simulink model "StateflowFactorial"  (R2016a)
settings: Solver=FixedStepDiscrete  StartTime=0.0  StopTime=10.0  RelTol=1e-3
settings Model: Creator=Mohamed Fawzy  LastModifiedBy=Mohamed Fawzy
settings OptimizationCC: DefaultParameterBehavior=Inlined  OptimizeModelRefInitCode=on  LifeSpan=1
settings RTWCC: SystemTargetFile=ert.tlc  GenCodeOnly=on  GenerateMakefile=off  TemplateMakefile=ert_default_tmf  GenerateReport=on  IncludeHyperlinkInReport=on  LaunchReport=on  GenerateTraceInfo=on  GenerateTraceReport=on  GenerateTraceReportSl=on  GenerateTraceReportSf=on  GenerateTraceReportEml=on
settings CodeAppCC: ForceParamTrailComments=on  IgnoreCustomStorageClasses=off  OperatorAnnotations=on  SimulinkDataObjDesc=on  SFDataObjDesc=on  MATLABFcnDesc=on  InsertBlockDesc=on  MATLABSourceComments=on
settings ERTTargetCC: GenerateSampleERTMain=on  SuppressErrorStatus=on  InlinedParameterPlacement=NonHierarchical  ERTCustomFileTemplate=example_file_process.tlc

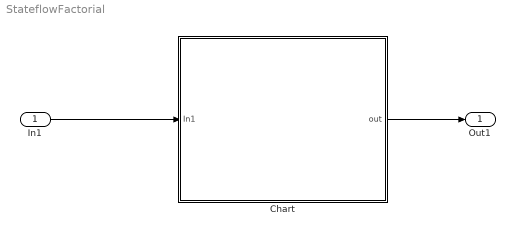
== system StateflowFactorial ==
  In1 : Inport  OutDataTypeStr=uint8
  Chart : Stateflow chart  TreatAsAtomicUnit=on
  Out1 : Outport  OutDataTypeStr=double
  wires:
  In1/1 -> Chart/1(In1)
  Chart/1(out) -> Out1/1

== stateflow chart StateflowFactorial/Chart ==
  (default) -> (junction 24) : % Factorial
  (junction 25) -> (junction 23) [order 1] : [i>0]
  (junction 23) -> (junction 26) : {out=out*i;}
  (junction 24) -> (junction 25) : {
      | out=1;
      | i=In1;
      | }
  (junction 26) -> (junction 25) : {i--;}
  (junction 25) -> (junction 27) [order 2]
  data: In1 input uint8; out output double; i local uint8
